simulink model "FP_PMSM_ProposedDTC"  (R2023b)
settings: Solver=ode1  StartTime=0.0  StopTime=2  FixedStep=140e-6  RelTol=1e-3
undefined symbols (not defined in the file): J, Lamda_PM, Lls, Ls, Mod_Lamda_s_ref, P, Rs
libraries: spsPWMGeneratorDCDCLib x1, spspowerguiLib x1
(part 2 of 2)

== matlab function FP_PMSM_ProposedDTC/Controller/Twenty Sectors code ==
  data: theta input; sector output
function sector = fcn(theta)
if(theta>0 && theta<=pi/10)
    sector=1;
elseif(theta>pi/10 && theta<=2*pi/10)
    sector=2;
elseif(theta>2*pi/10 && theta<=3*pi/10)
    sector=3;
elseif(theta>3*pi/10 && theta<=4*pi/10)
    sector=4;
elseif(theta>4*pi/10 && theta<=5*pi/10)
    sector=5;
elseif(theta>5*pi/10 && theta<=6*pi/10)
    sector=6;
elseif(theta>6*pi/10 && theta<=7*pi/10)
    sector=7;
elseif(theta>7*pi/10 && theta<=8*pi/10)
    sector=8;
elseif(theta>8*pi/10 && theta<=9*pi/10)
    sector=9;        
elseif(theta>9*pi/10 && theta<=pi)
    sector=10;
elseif(theta>-pi && theta<=-9*pi/10)
    sector=11;
elseif(theta>-9*pi/10 && theta<=-8*pi/10)
    sector=12;
elseif(theta>-8*pi/10 && theta<=-7*pi/10)
    sector=13;
elseif(theta>-7*pi/10 && theta<=-6*pi/10)
    sector=14;
elseif(theta>-6*pi/10 && theta<=-5*pi/10)
    sector=15;
elseif(theta>-5*pi/10 && theta<=-4*pi/10)
    sector=16;
elseif(theta>-4*pi/10 && theta<=-3*pi/10)
    sector=17;
elseif(theta>-3*pi/10&& theta<=-2*pi/10)
    sector=18;
elseif(theta>-2*pi/10 && theta<=-pi/10)
    sector=19;
else
    sector=20;
end

== matlab function FP_PMSM_ProposedDTC/Controller/two samples ==
  data: Vt input; Vf input; V output

function V  = fcn(Vt,Vf)
persistent t1 x_opt
if isempty(t1),t1=0;end
if isempty(x_opt),x_opt=1;end
% Flux controlling voltage vector
if(mod(t1,2))==0
    x_opt=Vf;    
end 
% Torque controlling voltage vector
if(mod(t1,2))~=0
     x_opt=Vt;   
end
t1=t1+1;
V=x_opt;

== matlab function FP_PMSM_ProposedDTC/Controller/vector magnitude and angle/Vt and Vf in complex form ==
  data: Vt input; vt output; Vf input; vf output; Vdc input; thetaT output; thetaF output
function [vt,vf,thetaT,thetaF]  = fcn(Vt,Vf,Vdc)
vt=0;
vf=0;
thetaT=0;
thetaF=0;
% Torque controlling voltage vectors
if(Vt==0)
vt=abs(0);
thetaT=angle(0);
elseif(Vt==1)
vt=abs(2/5*Vdc*(1.6180+1j*0));
thetaT=angle(2/5*Vdc*(1.6180+1j*0));
elseif(Vt==2)
vt=abs(2/5*Vdc*(1.3090+1j*0.9511));
thetaT=angle(2/5*Vdc*(1.3090+1j*0.9511));
elseif(Vt==3)
vt=abs(2/5*Vdc*(0.5+1j*1.5390));
thetaT=angle(2/5*Vdc*(0.5+1j*1.5390));
elseif(Vt==4)
vt=abs(2/5*Vdc*(-0.5+1j*1.5390));
thetaT=angle(2/5*Vdc*(-0.5+1j*1.5390));
elseif(Vt==5)
vt=abs(2/5*Vdc*(-1.3090+1j*0.9511));
thetaT=angle(2/5*Vdc*(-1.3090+1j*0.9511));
elseif(Vt==6)
vt=abs(2/5*Vdc*(-1.6180+1j*0));
thetaT=angle(2/5*Vdc*(-1.6180+1j*0));
elseif(Vt==7)
vt=abs(2/5*Vdc*(-1.3090-1j*0.9511));
thetaT=angle(2/5*Vdc*(-1.3090-1j*0.9511));
elseif(Vt==8)
vt=abs(2/5*Vdc*(-0.5-1j*1.5390));
thetaT=angle(2/5*Vdc*(-0.5-1j*1.5390));
elseif(Vt==9)
vt=abs(2/5*Vdc*(0.5-1j*1.5390));
thetaT=angle(2/5*Vdc*(0.5-1j*1.5390));
elseif(Vt==10)
vt=abs(2/5*Vdc*(1.3090-1j*0.9511));
thetaT=angle(2/5*Vdc*(1.3090-1j*0.9511));
elseif(Vt==11)
vt=abs(2/5*Vdc*(1+1j*0));
thetaT=angle(2/5*Vdc*(1+1j*0));
elseif(Vt==12)
vt=abs(2/5*Vdc*(0.8090+1j*0.5878));
thetaT=angle(2/5*Vdc*(0.8090+1j*0.5878));
elseif(Vt==13)
vt=abs(2/5*Vdc*(0.3090+1j*0.9511));
thetaT=angle(2/5*Vdc*(0.3090+1j*0.9511));
elseif(Vt==14)
vt=abs(2/5*Vdc*(-0.3090+1j*0.9511));
thetaT=angle(2/5*Vdc*(-0.3090+1j*0.9511));
elseif(Vt==15)
vt=abs(2/5*Vdc*(-0.8090+1j*0.5878));
thetaT=angle(2/5*Vdc*(-0.8090+1j*0.5878));
elseif(Vt==16)
vt=abs(2/5*Vdc*(-1+1j*0));
thetaT=angle(2/5*Vdc*(-1+1j*0));
elseif(Vt==17)
vt=abs(2/5*Vdc*(-0.8090-1j*0.5878));
thetaT=angle(2/5*Vdc*(-0.8090-1j*0.5878));
elseif(Vt==18)
vt=abs(2/5*Vdc*(-0.3090-1j*0.9511));
thetaT=angle(2/5*Vdc*(-0.3090-1j*0.9511));
elseif(Vt==19)
vt=abs(2/5*Vdc*(0.3090-1j*0.9511));
thetaT=angle(2/5*Vdc*(0.3090-1j*0.9511));
elseif(Vt==20)
vt=abs(2/5*Vdc*(0.8090-1j*0.5878));
thetaT=angle(2/5*Vdc*(0.8090-1j*0.5878));
elseif(Vt==21)
vt=abs(2/5*Vdc*(0.6180+1j*0));
thetaT=angle(2/5*Vdc*(0.6180+1j*0));
elseif(Vt==22)
vt=abs(2/5*Vdc*(0.5+1j*0.3633));
thetaT=angle(2/5*Vdc*(0.5+1j*0.3633));
elseif(Vt==23)
vt=abs(2/5*Vdc*(0.1910+1j*0.5878));
thetaT=angle(2/5*Vdc*(0.1910+1j*0.5878));
elseif(Vt==24)
vt=abs(2/5*Vdc*(-0.1910+1j*0.5878));
thetaT=angle(2/5*Vdc*(-0.1910+1j*0.5878));
elseif(Vt==25)
vt=abs(2/5*Vdc*(-0.5+1j*0.3633));
thetaT=angle(2/5*Vdc*(-0.5+1j*0.3633));
elseif(Vt==26)
vt=abs(2/5*Vdc*(-0.6180+1j*0));
thetaT=angle(2/5*Vdc*(-0.6180+1j*0));
elseif(Vt==27)
vt=abs(2/5*Vdc*(-0.5-1j*0.3633));
thetaT=angle(2/5*Vdc*(-0.5-1j*0.3633));
elseif(Vt==28)
vt=abs(2/5*Vdc*(-0.1910-1j*0.5878));
thetaT=angle(2/5*Vdc*(-0.1910-1j*0.5878));
elseif(Vt==29)
vt=abs(2/5*Vdc*(0.1910-1j*0.5878));
thetaT=angle(2/5*Vdc*(0.1910-1j*0.5878));
elseif(Vt==30)
vt=abs(2/5*Vdc*(0.5-1j*0.3633));
thetaT=angle(2/5*Vdc*(0.5-1j*0.3633));
elseif(Vt==31)
vt=abs(0);
thetaT=angle(0);
end

% Flux controlling voltage vectors

if(Vf==0)
vf=abs(0);
thetaF=angle(0);
elseif(Vf==1)
vf=abs(2/5*Vdc*(1.6180+1j*0));
thetaF=angle(2/5*Vdc*(1.6180+1j*0));
elseif(Vf==2)
vf=abs(2/5*Vdc*(1.3090+1j*0.9511));
thetaF=angle(2/5*Vdc*(1.3090+1j*0.9511));
elseif(Vf==3)
vf=abs(2/5*Vdc*(0.5+1j*1.5390));
thetaF=angle(2/5*Vdc*(0.5+1j*1.5390));
elseif(Vf==4)
vf=abs(2/5*Vdc*(-0.5+1j*1.5390));
thetaF=angle(2/5*Vdc*(-0.5+1j*1.5390));
elseif(Vf==5)
vf=abs(2/5*Vdc*(-1.3090+1j*0.9511));
thetaF=angle(2/5*Vdc*(-1.3090+1j*0.9511));
elseif(Vf==6)
vf=abs(2/5*Vdc*(-1.6180+1j*0));
thetaF=angle(2/5*Vdc*(-1.6180+1j*0));
elseif(Vf==7)
vf=abs(2/5*Vdc*(-1.3090-1j*0.9511));
thetaF=angle(2/5*Vdc*(-1.3090-1j*0.9511));
elseif(Vf==8)
vf=abs(2/5*Vdc*(-0.5-1j*1.5390));
thetaF=angle(2/5*Vdc*(-0.5-1j*1.5390));
elseif(Vf==9)
vf=abs(2/5*Vdc*(0.5-1j*1.5390));
thetaF=angle(2/5*Vdc*(0.5-1j*1.5390));
elseif(Vf==10)
vf=abs(2/5*Vdc*(1.3090-1j*0.9511));
thetaF=angle(2/5*Vdc*(1.3090-1j*0.9511));
elseif(Vf==11)
vf=abs(2/5*Vdc*(1+1j*0));
thetaF=angle(2/5*Vdc*(1+1j*0));
elseif(Vf==12)
vf=abs(2/5*Vdc*(0.8090+1j*0.5878));
thetaF=angle(2/5*Vdc*(0.8090+1j*0.5878));
elseif(Vf==13)
vf=abs(2/5*Vdc*(0.3090+1j*0.9511));
thetaF=angle(2/5*Vdc*(0.3090+1j*0.9511));
elseif(Vf==14)
vf=abs(2/5*Vdc*(-0.3090+1j*0.9511));
thetaF=angle(2/5*Vdc*(-0.3090+1j*0.9511));
elseif(Vf==15)
vf=abs(2/5*Vdc*(-0.8090+1j*0.5878));
thetaF=angle(2/5*Vdc*(-0.8090+1j*0.5878));
elseif(Vf==16)
vf=abs(2/5*Vdc*(-1+1j*0));
thetaF=angle(2/5*Vdc*(-1+1j*0));
elseif(Vf==17)
vf=abs(2/5*Vdc*(-0.8090-1j*0.5878));
thetaF=angle(2/5*Vdc*(-0.8090-1j*0.5878));
elseif(Vf==18)
vf=abs(2/5*Vdc*(-0.3090-1j*0.9511));
thetaF=angle(2/5*Vdc*(-0.3090-1j*0.9511));
elseif(Vf==19)
vf=abs(2/5*Vdc*(0.3090-1j*0.9511));
thetaF=angle(2/5*Vdc*(0.3090-1j*0.9511));
elseif(Vf==20)
vf=abs(2/5*Vdc*(0.8090-1j*0.5878));
thetaF=angle(2/5*Vdc*(0.8090-1j*0.5878));
elseif(Vf==21)
vf=abs(2/5*Vdc*(0.6180+1j*0));
thetaF=angle(2/5*Vdc*(0.6180+1j*0));
elseif(Vf==22)
vf=abs(2/5*Vdc*(0.5+1j*0.3633));
thetaF=angle(2/5*Vdc*(0.5+1j*0.3633));
elseif(Vf==23)
vf=abs(2/5*Vdc*(0.1910+1j*0.5878));
thetaF=angle(2/5*Vdc*(0.1910+1j*0.5878));
elseif(Vf==24)
vf=abs(2/5*Vdc*(-0.1910+1j*0.5878));
thetaF=angle(2/5*Vdc*(-0.1910+1j*0.5878));
elseif(Vf==25)
vf=abs(2/5*Vdc*(-0.5+1j*0.3633));
thetaF=angle(2/5*Vdc*(-0.5+1j*0.3633));
elseif(Vf==26)
vf=abs(2/5*Vdc*(-0.6180+1j*0));
thetaF=angle(2/5*Vdc*(-0.6180+1j*0));
elseif(Vf==27)
vf=abs(2/5*Vdc*(-0.5-1j*0.3633));
thetaF=angle(2/5*Vdc*(-0.5-1j*0.3633));
elseif(Vf==28)
vf=abs(2/5*Vdc*(-0.1910-1j*0.5878));
thetaF=angle(2/5*Vdc*(-0.1910-1j*0.5878));
elseif(Vf==29)
vf=abs(2/5*Vdc*(0.1910-1j*0.5878));
thetaF=angle(2/5*Vdc*(0.1910-1j*0.5878));
elseif(Vf==30)
vf=abs(2/5*Vdc*(0.5-1j*0.3633));
thetaF=angle(2/5*Vdc*(0.5-1j*0.3633));
elseif(Vf==31)
vf=abs(0);
thetaF=angle(0);
end

== matlab function FP_PMSM_ProposedDTC/INVERTER/MATLAB Function ==
  data: Sa input; Van output; Sb input; Sc input; Sd input; Se input; Vdc input; Vbn output; Vcn output; Vdn output; Ven output
function [Van,Vbn,Vcn,Vdn,Ven]= fcn(Sa,Sb,Sc,Sd,Se,Vdc)
Van=(Vdc/5)*(4*Sa-Sb-Sc-Sd-Se);
Vbn=(Vdc/5)*(4*Sb-Sa-Sc-Sd-Se);
Vcn=(Vdc/5)*(4*Sc-Sa-Sb-Sd-Se);
Vdn=(Vdc/5)*(4*Sd-Sa-Sb-Sc-Se);
Ven=(Vdc/5)*(4*Se-Sa-Sb-Sc-Sd);

== matlab function FP_PMSM_ProposedDTC/Controller/Duty Application ==
  data: vv input; Sa output; Sb output; Sc output; Sd output; Se output; Dt input; Df input; Vopt output; D output

function [Sa,Sb,Sc,Sd,Se,Vopt,D] = fcn(vv,Dt,Df)
Sa=0;
Sb=0;
Sc=0;
Sd=0;
Se=0;
D=1;
persistent t1 x_opt
if isempty(t1),t1=0;end
if isempty(x_opt),x_opt=1;end
% Flux controlling voltage vector
if(mod(t1,2))==0
    D=Df;
    x_opt=vv;
    if(vv==0)
    Sa=0;
    Sb=0;
    Sc=0; 
    Sd=0;
    Se=0;
    elseif(vv==1)
    Sa=1;
    Sb=1;
    Sc=0; 
    Sd=0;
    Se=1;
    elseif(vv==2)
    Sa=1;
    Sb=1;
    Sc=0;
    Sd=0;
    Se=0;
    elseif(vv==3)
    Sa=1;
    Sb=1;
    Sc=1;
    Sd=0;
    Se=0;
    elseif(vv==4)
    Sa=0;
    Sb=1;
    Sc=1;
    Sd=0;
    Se=0;
    elseif(vv==5)
    Sa=0;
    Sb=1;
    Sc=1;
    Sd=1;
    Se=0;
    elseif(vv==6)
    Sa=0;
    Sb=0;
    Sc=1;
    Sd=1;
    Se=0;
    elseif(vv==7)
    Sa=0;
    Sb=0;
    Sc=1;
    Sd=1;
    Se=1;
    elseif(vv==8)
    Sa=0;
    Sb=0;
    Sc=0;
    Sd=1;
    Se=1;
    elseif(vv==9)
    Sa=1;
    Sb=0;
    Sc=0;
    Sd=1;
    Se=1;
    elseif(vv==10)
    Sa=1;
    Sb=0;
    Sc=0;
    Sd=0;
    Se=1;
    elseif(vv==11)
    Sa=1;
    Sb=0;
    Sc=0;
    Sd=0;
    Se=0;
    elseif(vv==12)
    Sa=1;
    Sb=1;
    Sc=1;
    Sd=0;
    Se=1;
    elseif(vv==13)
    Sa=0;
    Sb=1;
    Sc=0;
    Sd=0;
    Se=0;
    elseif(vv==14)
    Sa=1;
    Sb=1;
    Sc=1;
    Sd=1;
    Se=0;
    elseif(vv==15)
    Sa=0;
    Sb=0;
    Sc=1;
    Sd=0;
    Se=0;
    elseif(vv==16)
    Sa=0;
    Sb=1;
    Sc=1;
    Sd=1;
    Se=1;
    elseif(vv==17)
    Sa=0;
    Sb=0;
    Sc=0;
    Sd=1;
    Se=0;
    elseif(vv==18)
    Sa=1;
    Sb=0;
    Sc=1;
    Sd=1;
    Se=1;
    elseif(vv==19)
    Sa=0;
    Sb=0;
    Sc=0;
    Sd=0;
    Se=1;
    elseif(vv==20)
    Sa=1;
    Sb=1;
    Sc=0;
    Sd=1;
    Se=1;
    elseif(vv==21)
    Sa=0;
    Sb=1;
    Sc=0;
    Sd=0;
    Se=1;
    elseif(vv==22)
    Sa=1;
    Sb=1;
    Sc=0;
    Sd=1;
    Se=0;
    elseif(vv==23)
    Sa=1;
    Sb=0;
    Sc=1;
    Sd=0;
    Se=0;
    elseif(vv==24)
    Sa=0;
    Sb=1;
    Sc=1;
    Sd=0;
    Se=1;
    elseif(vv==25)
    Sa=0;
    Sb=1;
    Sc=0;
    Sd=1;
    Se=0;
    elseif(vv==26)
    Sa=1;
    Sb=0;
    Sc=1;
    Sd=1;
    Se=0;
    elseif(vv==27)
    Sa=0;
    Sb=0;
    Sc=1;
    Sd=0;
    Se=1;
    elseif(vv==28)
    Sa=0;
    Sb=1;
    Sc=0;
    Sd=1;
    Se=1;
    elseif(vv==29)
    Sa=1;
    Sb=0;
    Sc=0;
    Sd=1;
    Se=0;
    elseif(vv==30)
    Sa=1;
    Sb=0;
    Sc=1;
    Sd=0;
    Se=1;
    else
    Sa=1;
    Sb=1;
    Sc=1;
    Sd=1;
    Se=1;
    end
end
% Torque controlling voltage vector
if(mod(t1,2))~=0
    D=Dt;
     x_opt=vv;
    if(vv==0)
    Sa=0;
    Sb=0;
    Sc=0; 
    Sd=0;
    Se=0;
    elseif(vv==1)
    Sa=1;
    Sb=1;
    Sc=0;
    Sd=0;
    Se=1;
    elseif(vv==2)
    Sa=1;
    Sb=1;
    Sc=0;
    Sd=0;
    Se=0;
    elseif(vv==3)
    Sa=1;
    Sb=1;
    Sc=1;
    Sd=0;
    Se=0;
    elseif(vv==4)
    Sa=0;
    Sb=1;
    Sc=1;
    Sd=0;
    Se=0;
    elseif(vv==5)
    Sa=0;
    Sb=1;
    Sc=1;
    Sd=1;
    Se=0;
    elseif(vv==6)
    Sa=0;
    Sb=0;
    Sc=1;
    Sd=1;
    Se=0;
    elseif(vv==7)
    Sa=0;
    Sb=0;
    Sc=1;
    Sd=1;
    Se=1;
    elseif(vv==8)
    Sa=0;
    Sb=0;
    Sc=0;
    Sd=1;
    Se=1;
    elseif(vv==9)
    Sa=1;
    Sb=0;
    Sc=0;
    Sd=1;
    Se=1;
    elseif(vv==10)
    Sa=1;
    Sb=0;
    Sc=0;
    Sd=0;
    Se=1;
    elseif(vv==11)
    Sa=1;
    Sb=0;
    Sc=0;
    Sd=0;
    Se=0;
    elseif(vv==12)
    Sa=1;
    Sb=1;
    Sc=1;
    Sd=0;
    Se=1;
    elseif(vv==13)
    Sa=0;
    Sb=1;
    Sc=0;
    Sd=0;
    Se=0;
    elseif(vv==14)
    Sa=1;
    Sb=1;
    Sc=1;
    Sd=1;
    Se=0;
    elseif(vv==15)
    Sa=0;
    Sb=0;
    Sc=1;
    Sd=0;
    Se=0;
    elseif(vv==16)
    Sa=0;
    Sb=1;
    Sc=1;
    Sd=1;
    Se=1;
    elseif(vv==17)
    Sa=0;
    Sb=0;
    Sc=0;
    Sd=1;
    Se=0;
    elseif(vv==18)
    Sa=1;
    Sb=0;
    Sc=1;
    Sd=1;
    Se=1;
    elseif(vv==19)
    Sa=0;
    Sb=0;
    Sc=0;
    Sd=0;
    Se=1;
    elseif(vv==20)
    Sa=1;
    Sb=1;
    Sc=0;
    Sd=1;
    Se=1;
    elseif(vv==21)
    Sa=0;
    Sb=1;
    Sc=0;
    Sd=0;
    Se=1;
    elseif(vv==22)
    Sa=1;
    Sb=1;
    Sc=0;
    Sd=1;
    Se=0;
    elseif(vv==23)
    Sa=1;
    Sb=0;
    Sc=1;
    Sd=0;
    Se=0;
    elseif(vv==24)
    Sa=0;
    Sb=1;
    Sc=1;
    Sd=0;
    Se=1;
    elseif(vv==25)
    Sa=0;
    Sb=1;
    Sc=0;
    Sd=1;
    Se=0;
    elseif(vv==26)
    Sa=1;
    Sb=0;
    Sc=1;
    Sd=1;
    Se=0;
    elseif(vv==27)
    Sa=0;
    Sb=0;
    Sc=1;
    Sd=0;
    Se=1;
    elseif(vv==28)
    Sa=0;
    Sb=1;
    Sc=0;
    Sd=1;
    Se=1;
    elseif(vv==29)
    Sa=1;
    Sb=0;
    Sc=0;
    Sd=1;
    Se=0;
    elseif(vv==30)
    Sa=1;
    Sb=0;
    Sc=1;
    Sd=0;
    Se=1;
    else
    Sa=1;
    Sb=1;
    Sc=1;
    Sd=1;
    Se=1;
    end
end
t1=t1+1;
Vopt=x_opt;

== matlab function FP_PMSM_ProposedDTC/Controller/Harmonic sector  ==
  data: theta input; sector output
function sector = fcn(theta)
if(theta>-pi/10 && theta<=pi/10)
    sector=1;
elseif(theta>pi/10 && theta<=3*pi/10)
    sector=2;
elseif(theta>3*pi/10 && theta<=pi/2)
    sector=3;
elseif(theta>pi/2 && theta<=7*pi/10)
    sector=4;
elseif(theta>7*pi/10 && theta<=9*pi/10)
    sector=5;
elseif(theta>-9*pi/10 && theta<=-7*pi/10)
    sector=7;
elseif(theta>-7*pi/10 && theta<=-pi/2)
    sector=8;
elseif(theta>-pi/2 && theta<=-3*pi/10)
    sector=9;
elseif(theta>-3*pi/10 && theta<=-pi/10)
    sector=10;        
else
    sector=6;
end
